simulink model "sl_rrmc2"  (R2022a)
settings: Solver=ode45  StartTime=0.0  StopTime=10.0  RelTol=1e-3  EnableMultiTasking=on
PreLoadFcn:
  | % Load PUMA robot, so it's available for manipulator blocks
  | if ~exist("puma","var") || ~exist("conf","var")
  |    [puma,conf] = loadrvcrobot("puma");
  | end
InitFcn:
  | if ~exist("puma","var") || ~exist("conf","var")
  |    [puma,conf] = loadrvcrobot("puma");
  | end
undefined symbols (not defined in the file or in its folder): conf, DiscIntNeverNeededParam, puma, se3, trvec2tform
libraries: robotcorelib x2, robotmaniplib x2, roblocks x1
settings Model: ExtModeTrigMode=oneshot  ExtModeArmWhenConnect=off  Creator=pic  LastModifiedBy=rpill
settings SolverCC: AlgebraicLoopSolver=TrustRegion  MaxZcPerStep=1
settings DataIOCC: SaveFormat=Array  SignalLoggingSaveFormat=ModelDataLogs  ReturnWorkspaceOutputs=off
settings OptimizationCC: BlockReduction=off  BooleanDataType=off  ExpressionDepthLimit=2147483647  InitFltsAndDblsToZero=on  LifeSpan=inf
settings DebuggingCC: SaveWithParameterizedLinksMsg=none  UnderspecifiedInitializationDetection=Classic  MergeDetectMultiDrivingBlocksExec=none  SignalResolutionControl=TryResolveAllWithWarning  MultiTaskDSMMsg=warning  MultiTaskCondExecSysMsg=none  FcnCallInpInsideContextMsg=warning  UnconnectedInputMsg=warning  UnconnectedOutputMsg=warning  UnconnectedLineMsg=warning  AllowSymbolicDim=off  StateNameClashWarn=warning  SFUnexpectedBacktrackingDiag=warning  SFNoUnconditionalDefaultTransitionDiag=warning  SFExecutionAtInitializationDiag=none  SFMachineParentedDataDiag=warning  ArithmeticOperatorsInVariantConditions=warning
settings HardwareCC: ProdBitPerPointer=32  ProdBitPerSizeT=32  ProdBitPerPtrDiffT=32  ProdLargestAtomicFloat=None  ProdIntDivRoundTo=Undefined  ProdEndianess=Unspecified  ProdWordSize=32  ProdHWDeviceType=32-bit Generic  TargetBitPerPointer=64  TargetBitPerSizeT=64  TargetBitPerPtrDiffT=64  TargetLongLongMode=on  TargetIntDivRoundTo=Zero  TargetEndianess=LittleEndian  TargetWordSize=64  TargetHWDeviceType=MATLAB Host  ProdEqTarget=off
settings ModelReferenceCC: PropagateSignalLabelsOutOfModel=off
settings SFSimCC: SimUseLocalCustomCode=off  CustomCodeUndefinedFunction=UseInterfaceOnly
settings RTWCC: RTWUseLocalCustomCode=off  DLArmComputeVersion=19.05
settings CodeAppCC: StateflowObjectComments=on
settings GRTTargetCC: TargetLangStandard=C89/C90 (ANSI)  ModelReferenceCompliant=off  CompOptLevelCompliant=off  CombineOutputUpdateFcns=off  MatFileLogging=off  GRTInterface=on
settings ConfigComp: CovMetricSettings=dw  CovSaveCumulativeToWorkspaceVar=on  CovSaveSingleToWorkspaceVar=on  CovExternalEMLEnable=off

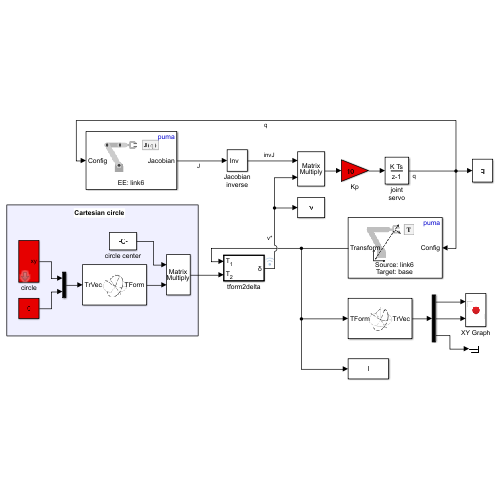
[thumbnail: Simulink's stored preview of the top-level diagram]
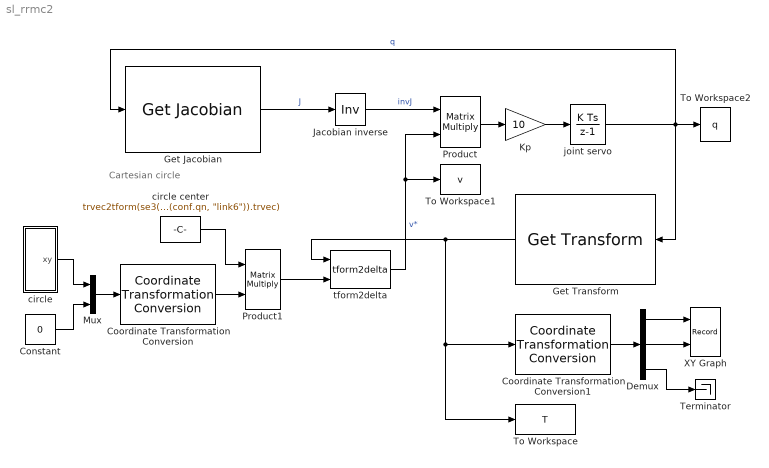
== system sl_rrmc2 ==
  note: Cartesian circle
  Constant : Constant  Value=0
  Coordinate Transformation Conversion : robotcorelib/Coordinate Transformation Conversion  InputRepresentation=Translation Vector  InputEulerSequence=ZYX  ShowTrVecInputPort=on  OutputRepresentation=Homogeneous Transformation  OutputEulerSequence=ZYX  ShowTrVecOutputPort=on  SimulateUsing=Interpreted execution
      settings: SourceProductBaseCode=NV,RO,RR,UV
  Coordinate Transformation Conversion1 : robotcorelib/Coordinate Transformation Conversion  InputRepresentation=Homogeneous Transformation  InputEulerSequence=ZYX  ShowTrVecInputPort=on  OutputRepresentation=Translation Vector  OutputEulerSequence=ZYX  ShowTrVecOutputPort=on  SimulateUsing=Interpreted execution
      settings: SourceProductBaseCode=NV,RO,RR,UV
  Demux : Demux  Outputs=3
  Get Jacobian : robotmaniplib/Get Jacobian  RigidBodyTree=puma  EndEffector=link6  SimulateUsing=Interpreted execution
      settings: SourceProductBaseCode=RO
  Get Transform : robotmaniplib/Get Transform  RigidBodyTree=puma  SourceBody=link6  TargetBody=base  SimulateUsing=Interpreted execution
  Jacobian inverse : Product  Inputs=/  Multiplication=Matrix(*)
  Kp : Gain  Gain=10  SaturateOnIntegerOverflow=on  OutDataTypeStr=Inherit: Same as input  ParamDataTypeStr=Inherit: Same as input
  Mux : Mux  Inputs=2
  Product : Product  Multiplication=Matrix(*)  InputSameDT=on  RndMeth=Zero  SaturateOnIntegerOverflow=on  OutDataTypeStr=Inherit: Same as first input
  Product1 : Product  Multiplication=Matrix(*)  InputSameDT=on  RndMeth=Zero  SaturateOnIntegerOverflow=on  OutDataTypeStr=Inherit: Same as first input
  Terminator : Terminator
  To Workspace : ToWorkspace  VariableName=T  SampleTime=-1
  To Workspace1 : ToWorkspace  VariableName=v  SampleTime=-1
  To Workspace2 : ToWorkspace  VariableName=q  SampleTime=-1
  XY Graph : Record  FileSettingsInternal="{\"entries\":[{\"content\":{\"excelSettings\":{\"content\":{},\"type\":\"Streamout.ExcelSettings\"}},\"type\":\"Streamout.FileSettingStorage\",\"uuid\":\"0d20cd93-21cb-4002-bd40-8dafefab4146\"}],\"packageUris\":[\"http://schema.mathworks.com/mf0/streamout_blocks/R2020a\"],\"version\":\"1.0\"}"  Layout=[1 1]  SignalsInternal="{\"entries\":[{\"content\":{\"signals\":[{\"content\":{\"blockPath\":[\"sl_rrmc2/XY Graph\"],\"channel\":[],\"dimensions\":[1,1],\"domain\":\"sl_rrmc2/XY Graph\",\"lineColor\":\"#a2142f\",\"plots\":[1],\"port\":1,\"sid\":[],\"signalID\":32,\"signalName\":\"Demux:1\"},\"type\":\"RecordBlkView.Signal\",\"uuid\":\"7985a69c-e644-418d-880d-7244cf26725e\"},{\"content\":{\"blockPath\":[\"sl_rrmc2/XY Graph\"],\"channel\":[],\"dimensions\":[1,1],\"domain\":\"sl_rrmc2/XY Graph\",\"lineColor\":\"#139fff\",\"plots\":[1],\"port\":2,\"sid\":[],\"signalID\":35,\"signalName\":\"Demux:2\"},\"type\":\"RecordBlkView.Signal\",\"uuid\":\"68fb1052-2366-4f23-abdc-8ecbcf043e07\"}]},\"type\":\"RecordBlkView.InputSignals\",\"uuid\":\"898e0df4-c276-4478-894c-db8fc82ed8b5\"}],\"packageUris\":[\"http://schema.mathworks.com/mf0/streamout_blocks/R2020a\"],\"version\":\"1.0\"}"  VisualizationBindings="{\"xyplotplugin\":{\"info\":[{\"series\":[{\"bindingParametersList\":[{\"parameter\":\"X-Axis\",\"signalID\":32,\"signalName\":\"Demux:1\"},{\"parameter\":\"Y-Axis\",\"signalID\":35,\"signalName\":\"Demux:2\"}],\"seriesID\":14674}],\"subplotID\":1}]}}"  CompatibilityTag=XY  st=-1
  circle : Subsystem  mask{radius=0.05, freq=0.2}
      mask prompts: freq "Frequency (rev/s)"
  circle center : Constant  Value="trvec2tform(se3(puma.getTransform(conf.qn, \"link6\")).trvec)"
  joint servo : DiscreteIntegrator  InitialCondition=conf.qn'  SampleTime=0.05  ICPrevOutput=DiscIntNeverNeededParam  ICPrevScaledInput=DiscIntNeverNeededParam
  tform2delta : roblocks/tform2delta  SystemSampleTime=-1  VariantActivationTime=update diagram  Latency=0  AutoFrameSizeCalculation=off
  wires:
  joint servo/1 -> Get Jacobian/1, To Workspace2/1, Get Transform/1  "q"
  Demux/1 -> XY Graph/1
  Demux/2 -> XY Graph/2
  tform2delta/1 -> Product/2, To Workspace1/1  "v*"
  Get Jacobian/1 -> Jacobian inverse/1  "J"
  Product/1 -> Kp/1
  Jacobian inverse/1 -> Product/1  "invJ"
  Kp/1 -> joint servo/1
  circle/1(xy) -> Mux/1
  Constant/1 -> Mux/2
  Get Transform/1 -> To Workspace/1, Coordinate Transformation Conversion1/1, tform2delta/1
  Coordinate Transformation Conversion/1 -> Product1/2
  circle center/1 -> Product1/1
  Demux/3 -> Terminator/1
  Product1/1 -> tform2delta/2
  Mux/1 -> Coordinate Transformation Conversion/1
  Coordinate Transformation Conversion1/1 -> Demux/1

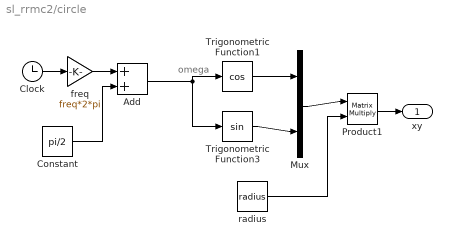
== system sl_rrmc2/circle ==
  note: omega
  Add : Sum
  Clock : Clock
  Constant : Constant  Value=pi/2
  Mux : Mux  Inputs=2
  Product1 : Product  Multiplication=Matrix(*)  RndMeth=Zero
  Trigonometric Function1 : Trigonometry  Operator=cos
  Trigonometric Function3 : Trigonometry
  freq : Gain  Gain=freq*2*pi
  radius : Constant  Value=radius
  xy : Outport
  wires:
  Add/1 -> Trigonometric Function1/1, Trigonometric Function3/1
  Product1/1 -> xy/1
  Clock/1 -> freq/1
  radius/1 -> Product1/2
  Mux/1 -> Product1/1
  Trigonometric Function1/1 -> Mux/1
  Trigonometric Function3/1 -> Mux/2
  freq/1 -> Add/1
  Constant/1 -> Add/2
